simulink model "System_franare"  (R2020b)
settings: Solver=ode45  StartTime=0.0  StopTime=15  FixedStep=0.00001  RelTol=1e-3
values from neighbouring files (symbols this model uses):
  Ar = eval(Ar)    [liniarizare_hydraulic_stud.m]
  Br = eval(Br)    [liniarizare_hydraulic_stud.m]
  C = [1 0 0 0 0]    [liniarizare_hydraulic_stud.m]
  K = place(Ar,Br,[-99  -100  -101  -200  -201])    [liniarizare_hydraulic_stud.m]
  L = L'    [liniarizare_hydraulic_stud.m]
  N = -inv(C*inv(Ar-Br*K)*Br)    [liniarizare_hydraulic_stud.m]
undefined symbols (not defined in the file or in its folder): proces, proces2
libraries: simulink x1
settings Model: Creator=Zsofi  LastModifiedBy=tudor
settings DataIOCC: ReturnWorkspaceOutputs=off
settings DebuggingCC: ArithmeticOperatorsInVariantConditions=warning
settings SFSimCC: SimUseLocalCustomCode=off  CustomCodeUndefinedFunction=UseInterfaceOnly
settings RTWCC: RTWUseLocalCustomCode=off
settings CodeAppCC: StateflowObjectComments=on

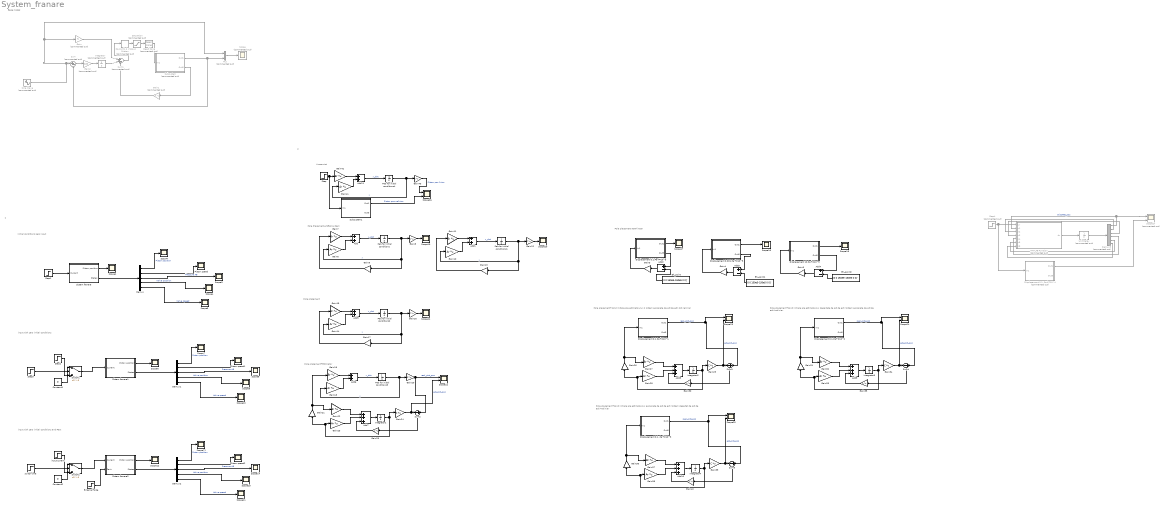
== system System_franare ==
  note: Linear sist
  note: Pole placement+cond initiale ale estimatorului si sistem apropiate de pct de ech sist neliniar
  note: 2
  note: Pole placement+Estimator
  note: Pole placement
  note: 1
  note: Pole Placement-LINEAR system
  note: input with zero initial conditions
  note: Initial conditions,zero input
  note: Base model
  note: input with zero initial conditions and Fext
  note: Pole placement NON-linear
  note: Pole placement+cond initiale ale estimatorului departate de pct de ech (sistem apropiate de pct de ech)-neliniar
  note: Pole placement+cond initiale ale estimatorului apropiate de pct de ech (sistem departat de pct de ech)-neliniar
  Add{,1,5..6,11} (5 alike) : Sum
  Add{7..10} (4 alike) : Sum  Inputs=+++
  Add2 : Sum  Inputs=+-
  Add3 : Sum  Inputs=+-
  Add4 : Sum  Inputs=+-
  Constant1 : Constant  Value=0
  Constant2 : Constant  Value=0
  Coulomb & Viscous Friction : simulink/Discontinuities/Coulomb & Viscous Friction  Commented=on  offset=0.005  gain=1
  DIsplacement 0.1,,Pa+=10^3 : Subsystem
  DIsplacement 0.1,,Pa+=10^4 : Subsystem  Commented=on
  DIsplacement 0.1,Pa+=10^1 : Subsystem
  DIsplacement 0.1,Pa+=10^2 : Subsystem
  DIsplacement 0.1,Pa+=10^5 : Subsystem
  Dead Zone : DeadZone  Commented=on  LowerValue=-0.005  UpperValue=0.005  SaturateOnIntegerOverflow=on
  Demux : Demux  Outputs=5
  Demux1 : Demux  Outputs=5
  Demux2 : Demux  Outputs=5
  Demux3 : Demux  Commented=on  Outputs=6
  Displacement 0.001,Pa+=10^5 : Subsystem
  Displacement 10,Pa+=10^5 : Subsystem
  Eh_point : Constant  Value=[0 0 150e5-150e5 0 0]'
  Eh_point1 : Constant  Value=[0 0 150e5-150e5 0 0]'
  Eh_point2 : Constant  Value=[0 0 150e5-150e5 0 0]'
  External force : Step  Time=6  After=300  SampleTime=0
  Gain : Gain  Commented=on  Gain=N
  Gain1 : Gain  Commented=on  Gain=K  Multiplication=Matrix(K*u)
  Gain{6,10,14,18,23,28,33,38,41} (9 alike) : Gain  Gain=Ar  Multiplication=Matrix(K*u)
  Gain{7,11,15,19,22,27,32,37,42} (9 alike) : Gain  Gain=Br  Multiplication=Matrix(K*u)
  Gain{8,12,16,20,24,29,34,39,43} (9 alike) : Gain  Gain=C  Multiplication=Matrix(K*u)
  Gain{3..5,9,13,17,21,26,31,36} (10 alike) : Gain  Gain=-K  Multiplication=Matrix(K*u)
  Gain2 : Gain  Commented=on  Gain=100
  Gain{25,30,35,40} (4 alike) : Gain  Gain=L  Multiplication=Matrix(K*u)
  Integrator : Integrator  Commented=on
  Integrator1 : Integrator
  Integrator2 : Integrator  InitialCondition=[0.01 0 0 0 0]'
  Integrator3 : Integrator  InitialCondition=[1 0 10e5 0 0]'
  Integrator4 : Integrator  InitialCondition=[0.4 0 1e5 0 0]'
  MATLAB Function : MATLAB Function  Commented=on  TreatAsAtomicUnit=on
  Mux : Mux  Commented=on  Inputs=2
  Pab for initial conditions : Integrator  InitialCondition=[0.1 0 1e5 0 0]
  Pab for initial conditions1 : Integrator  InitialCondition=[10 0 1e5 0 0]
  Pab for initial conditions2 : Integrator  InitialCondition=[0.1 0 1e5 0 0]
  Pab for initial conditions3 : Integrator  InitialCondition=[0.1 0 1e5 0 0]
  Pab for initial conditions4 : Integrator  InitialCondition=[0.001 0 0 0 0]
  Piston speed : Scope
  Piston speed1 : Scope
  Piston speed2 : Scope
  Saturation : Saturate  Commented=on  UpperLimit=0.1  LowerLimit=-0.1
  Scope : Scope  Commented=on
  Scope{1..21} (21 alike) : Scope
  Scope{22..26} (5 alike) : Scope  NumInputPorts=2
  Scope27 : Scope  Commented=on  NumInputPorts=2
  Sine Wave : Sin  Commented=on  Amplitude=0.02  Frequency=0.5  SampleTime=0
  Sistem franare : Subsystem
  Sistem franare1 : Subsystem
  Sistem franare2 : Subsystem
  Step : Step  Before=0.05  After=0  SampleTime=0
  Step1 : Step  Time=0  After=0  SampleTime=0
  Step2 : Step  Time=0  After=0.05  SampleTime=0
  Step3 : Step  SampleTime=0
  Step4 : Step  Commented=on  Time=0  After=0  SampleTime=0.00001
  Subsystem : Subsystem  Commented=on
  Subsystem1 : Subsystem
  Sum : Sum  Commented=on  Inputs=|+-
  Sum1 : Sum  Commented=on  Inputs=|++-
  Sum{2..5} (4 alike) : Sum  Inputs=-|+
  Switch1 : Switch  Criteria=u2 > Threshold
  Switch2 : Switch  Criteria=u2 > Threshold
  Unit Delay : UnitDelay  Commented=on  InitialCondition=[0.001 0 151e5 150e5 0 0]  SampleTime=-1  HasFrameUpgradeWarning=on
  input current : Step  Time=0  After=0.05  SampleTime=0
  switch time : Step  SampleTime=0
  wires:
  Subsystem/1(Out1) -> Mux/2, Sum/2
  Subsystem/2(Out3) -> Gain1/1
  Gain1/1 -> Sum1/3
  Sine Wave/1 -> Gain/1, Mux/1, Sum/1
  Gain/1 -> Sum1/1
  Sum/1 -> Gain2/1
  Gain2/1 -> Integrator/1
  Integrator/1 -> Sum1/2
  Mux/1 -> Scope/1
  Sum1/1 -> Coulomb & Viscous Friction/1
  Saturation/1 -> Dead Zone/1
  Dead Zone/1 -> Subsystem/1(In1)
  Coulomb & Viscous Friction/1 -> Saturation/1
  Sistem franare/1(Piston position) -> Scope1/1
  Sistem franare/2(States) -> Demux/1
  Demux/1 -> Scope2/1  "Piston position"
  Demux/2 -> Piston speed/1
  Demux/3 -> Scope3/1  "Pressure AB"
  Demux/4 -> Scope4/1  "Valve position"
  Demux/5 -> Scope5/1  "Valve speed"
  Step1/1 -> Sistem franare/1(Current)
  Step2/1 -> Switch1/3
  Demux1/2 -> Piston speed1/1
  Switch1/1 -> Sistem franare1/1(Current)
  Demux1/5 -> Scope10/1  "Valve speed"
  Sistem franare1/2(States) -> Demux1/1
  Demux1/4 -> Scope9/1  "Valve position"
  Constant1/1 -> Switch1/1
  Demux1/3 -> Scope8/1  "Pressure AB"
  Step3/1 -> Switch1/2
  Demux1/1 -> Scope7/1  "Piston position"
  Sistem franare1/1(Piston position) -> Scope6/1
  input current/1 -> Switch2/3
  Sistem franare2/2(States) -> Demux2/1
  Demux2/2 -> Piston speed2/1
  Switch2/1 -> Sistem franare2/1(Current)
  Demux2/5 -> Scope11/1  "Valve speed"
  Demux2/1 -> Scope13/1  "Piston position"
  Sistem franare2/1(Piston position) -> Scope12/1
  Constant2/1 -> Switch2/1
  Demux2/4 -> Scope15/1  "Valve position"
  switch time/1 -> Switch2/2
  Demux2/3 -> Scope14/1  "Pressure AB"
  External force/1 -> Sistem franare2/2(Fext)
  Displacement 0.001,Pa+=10^5/1(Out1) -> Scope16/1
  Gain4/1 -> Displacement 0.001,Pa+=10^5/1(In1)
  DIsplacement 0.1,Pa+=10^5/1(Out1) -> Scope17/1
  Gain3/1 -> DIsplacement 0.1,Pa+=10^5/1(In1)
  Displacement 10,Pa+=10^5/1(Out1) -> Scope18/1
  Gain5/1 -> Displacement 10,Pa+=10^5/1(In1)
  Pab for initial conditions/1 -> Gain8/1, Gain9/1, Gain6/1  "x"
  Gain6/1 -> Add/2
  Gain7/1 -> Add/1
  Add/1 -> Pab for initial conditions/1  "x_dot"
  Gain9/1 -> Gain7/1
  Gain8/1 -> Scope19/1
  Gain10/1 -> Add1/2
  Add1/1 -> Pab for initial conditions1/1  "x_dot"
  Gain13/1 -> Gain11/1
  Pab for initial conditions1/1 -> Gain12/1, Gain13/1, Gain10/1  "x"
  Gain11/1 -> Add1/1
  Gain12/1 -> Scope20/1
  Add2/1 -> Gain3/1
  DIsplacement 0.1,Pa+=10^5/2(Out3) -> Add2/1
  Eh_point/1 -> Add2/2
  Displacement 0.001,Pa+=10^5/2(Out3) -> Add3/1
  Eh_point1/1 -> Add3/2
  Add3/1 -> Gain4/1
  Displacement 10,Pa+=10^5/2(Out3) -> Add4/1
  Add4/1 -> Gain5/1
  Eh_point2/1 -> Add4/2
  Gain15/1 -> Add5/1
  Add5/1 -> Pab for initial conditions2/1  "x_dot"
  Gain16/1 -> Scope21/1
  Gain17/1 -> Gain15/1
  Gain14/1 -> Add5/2
  Pab for initial conditions2/1 -> Gain16/1, Gain17/1, Gain14/1  "x"
  Gain19/1 -> Add6/1
  Add6/1 -> Pab for initial conditions3/1  "x_dot"
  Gain20/1 -> Sum2/2, Scope22/1  "real_pist_pos"
  Gain21/1 -> Gain22/1, Gain19/1
  Gain18/1 -> Add6/2
  Pab for initial conditions3/1 -> Gain20/1, Gain18/1  "x"
  Gain23/1 -> Add7/2
  Gain22/1 -> Add7/1
  Gain24/1 -> Scope22/2, Sum2/1  "est_pist_pos"
  Add7/1 -> Integrator1/1
  Integrator1/1 -> Gain24/1, Gain21/1, Gain23/1
  Sum2/1 -> Gain25/1
  Gain25/1 -> Add7/3
  Sum3/1 -> Gain30/1
  Gain29/1 -> Scope23/2, Sum3/1  "est_pist_pos"
  Gain28/1 -> Add8/2
  Add8/1 -> Integrator2/1
  Gain30/1 -> Add8/3
  Gain27/1 -> Add8/1
  Gain26/1 -> DIsplacement 0.1,Pa+=10^1/1(In1), Gain27/1
  Integrator2/1 -> Gain29/1, Gain26/1, Gain28/1
  DIsplacement 0.1,Pa+=10^1/1(Out1) -> Scope23/1, Sum3/2  "real_pist_pos"
  DIsplacement 0.1,Pa+=10^2/1(Out1) -> Scope24/1, Sum4/2  "real_pist_pos"
  Gain35/1 -> Add9/3
  Gain32/1 -> Add9/1
  Gain31/1 -> DIsplacement 0.1,Pa+=10^2/1(In1), Gain32/1
  Gain33/1 -> Add9/2
  Add9/1 -> Integrator3/1
  Sum4/1 -> Gain35/1
  Integrator3/1 -> Gain34/1, Gain31/1, Gain33/1
  Gain34/1 -> Scope24/2, Sum4/1  "est_pist_pos"
  Gain39/1 -> Scope25/2, Sum5/1  "est_pist_pos"
  Integrator4/1 -> Gain39/1, Gain36/1, Gain38/1
  Gain38/1 -> Add10/2
  Sum5/1 -> Gain40/1
  Gain36/1 -> DIsplacement 0.1,,Pa+=10^3/1(In1), Gain37/1
  Gain40/1 -> Add10/3
  Add10/1 -> Integrator4/1
  DIsplacement 0.1,,Pa+=10^3/1(Out1) -> Scope25/1, Sum5/2  "real_pist_pos"
  Gain37/1 -> Add10/1
  Add11/1 -> Pab for initial conditions4/1  "x_dot"
  Gain41/1 -> Add11/2
  Pab for initial conditions4/1 -> Gain41/1, Gain43/1  "x"
  Gain42/1 -> Add11/1
  Step/1 -> Subsystem1/1(In1), Gain42/1
  Gain43/1 -> Scope26/1  "Piston pos liniar"
  Subsystem1/1(Out1) -> Scope26/2  "Piston pos neliniar"
  DIsplacement 0.1,,Pa+=10^4/1(Out1) -> Scope27/2
  Unit Delay/1 -> Demux3/1
  Demux3/1 -> Scope27/1, MATLAB Function/2(x1)  "Discrete_pos"
  Demux3/5 -> MATLAB Function/6(x5)
  Demux3/6 -> MATLAB Function/7(x6)
  Step4/1 -> DIsplacement 0.1,,Pa+=10^4/1(In1), MATLAB Function/1(uv)
  Demux3/3 -> MATLAB Function/4(x3)
  Demux3/4 -> MATLAB Function/5(x4)
  Demux3/2 -> MATLAB Function/3(x2)
  MATLAB Function/1(dx) -> Unit Delay/1

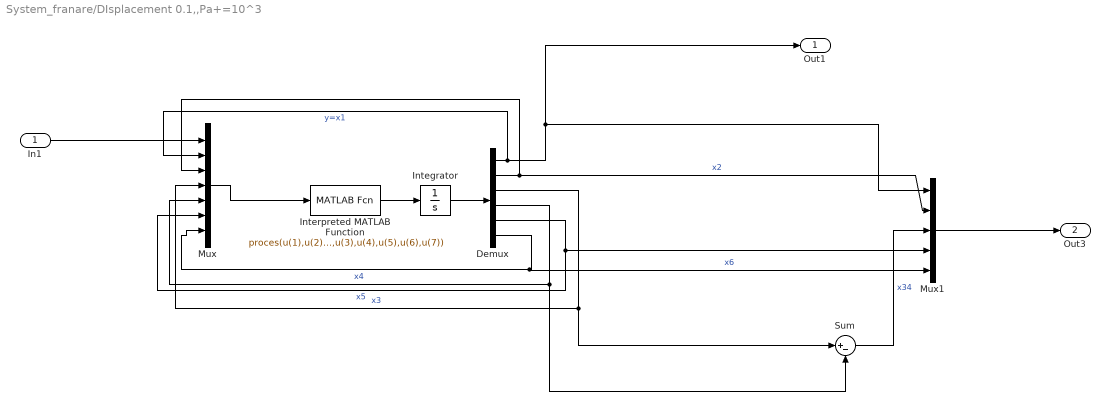
== system System_franare/DIsplacement 0.1,,Pa+=10^3 ==
  In1 : Inport
  Demux : Demux  Outputs=6
  Integrator : Integrator  InitialCondition=[1 0 150e5 150e5 0 0]
  Interpreted MATLAB Function : MATLABFcn  MATLABFcn=proces(u(1),u(2),u(3),u(4),u(5),u(6),u(7))  OutputSignalType=real  Output1D=off
  Mux : Mux  Inputs=7
  Mux1 : Mux  Inputs=5
  Sum : Sum  Inputs=|+-
  Out1 : Outport
  Out3 : Outport  Port=2
  wires:
  Demux/4 -> Sum/2, Mux/5  "x4"
  Demux/3 -> Sum/1, Mux/4  "x3"
  Demux/6 -> Mux1/5, Mux/7  "x6"
  Demux/5 -> Mux/6, Mux1/4  "x5"
  Demux/1 -> Mux/2, Out1/1, Mux1/1  "y=x1"
  Demux/2 -> Mux1/2, Mux/3  "x2"
  Interpreted MATLAB Function/1 -> Integrator/1
  In1/1 -> Mux/1
  Sum/1 -> Mux1/3  "x34"
  Integrator/1 -> Demux/1
  Mux1/1 -> Out3/1
  Mux/1 -> Interpreted MATLAB Function/1

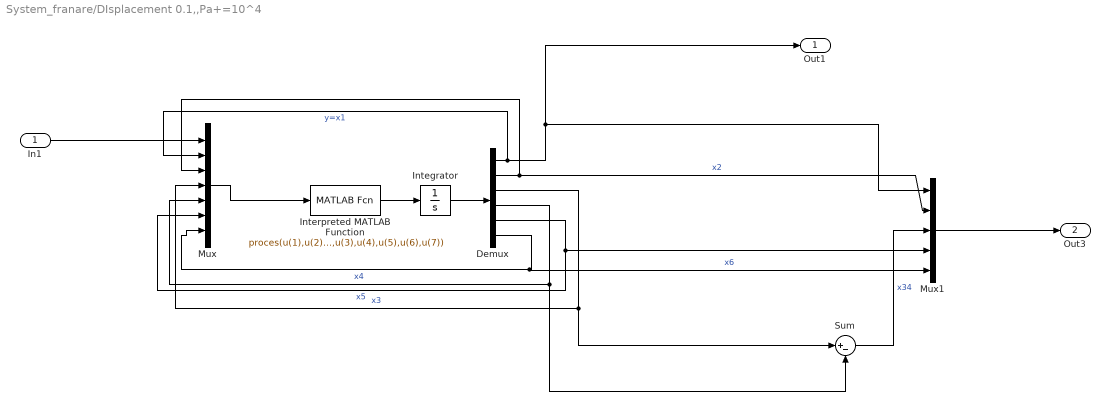
== system System_franare/DIsplacement 0.1,,Pa+=10^4 ==
  In1 : Inport
  Demux : Demux  Outputs=6
  Integrator : Integrator  InitialCondition=[0.001 0 151e5 150e5 0 0]
  Interpreted MATLAB Function : MATLABFcn  MATLABFcn=proces(u(1),u(2),u(3),u(4),u(5),u(6),u(7))  OutputSignalType=real  Output1D=off
  Mux : Mux  Inputs=7
  Mux1 : Mux  Inputs=5
  Sum : Sum  Inputs=|+-
  Out1 : Outport
  Out3 : Outport  Port=2
  wires:
  Demux/4 -> Sum/2, Mux/5  "x4"
  Demux/3 -> Sum/1, Mux/4  "x3"
  Demux/6 -> Mux1/5, Mux/7  "x6"
  Demux/5 -> Mux/6, Mux1/4  "x5"
  Demux/1 -> Mux/2, Out1/1, Mux1/1  "y=x1"
  Demux/2 -> Mux1/2, Mux/3  "x2"
  Interpreted MATLAB Function/1 -> Integrator/1
  In1/1 -> Mux/1
  Sum/1 -> Mux1/3  "x34"
  Integrator/1 -> Demux/1
  Mux1/1 -> Out3/1
  Mux/1 -> Interpreted MATLAB Function/1

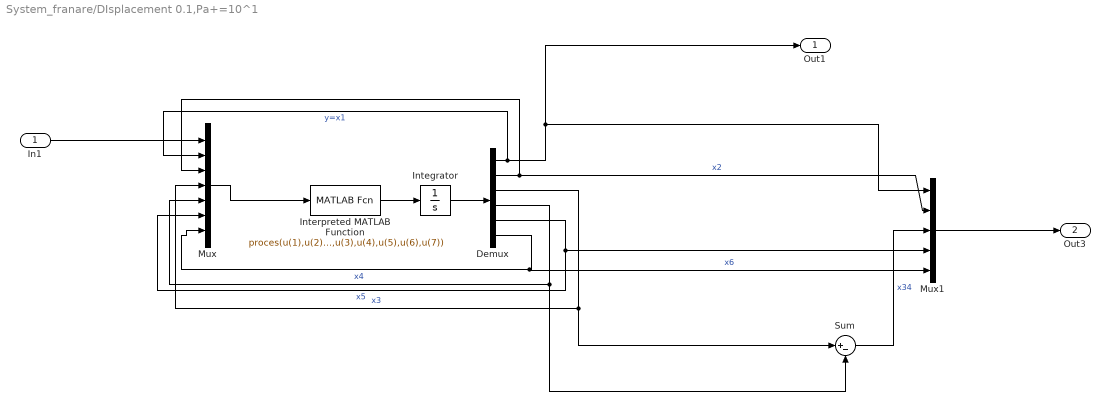
== system System_franare/DIsplacement 0.1,Pa+=10^1 ==
  In1 : Inport
  Demux : Demux  Outputs=6
  Integrator : Integrator  InitialCondition=[0.01 0 151e5 150e5 0 0]
  Interpreted MATLAB Function : MATLABFcn  MATLABFcn=proces(u(1),u(2),u(3),u(4),u(5),u(6),u(7))  OutputSignalType=real  Output1D=off
  Mux : Mux  Inputs=7
  Mux1 : Mux  Inputs=5
  Sum : Sum  Inputs=|+-
  Out1 : Outport
  Out3 : Outport  Port=2
  wires:
  Demux/4 -> Sum/2, Mux/5  "x4"
  Demux/3 -> Sum/1, Mux/4  "x3"
  Demux/6 -> Mux1/5, Mux/7  "x6"
  Demux/5 -> Mux/6, Mux1/4  "x5"
  Demux/1 -> Mux/2, Out1/1, Mux1/1  "y=x1"
  Demux/2 -> Mux1/2, Mux/3  "x2"
  Interpreted MATLAB Function/1 -> Integrator/1
  In1/1 -> Mux/1
  Sum/1 -> Mux1/3  "x34"
  Integrator/1 -> Demux/1
  Mux1/1 -> Out3/1
  Mux/1 -> Interpreted MATLAB Function/1

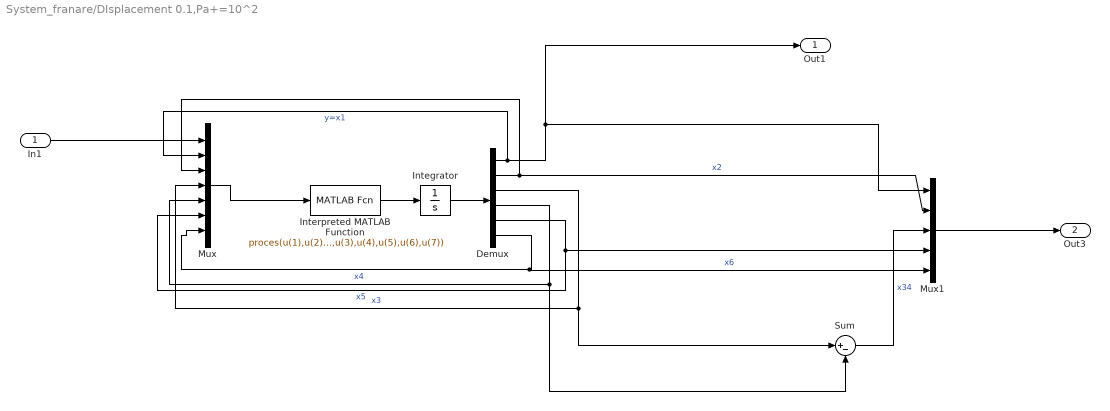
== system System_franare/DIsplacement 0.1,Pa+=10^2 ==
  In1 : Inport
  Demux : Demux  Outputs=6
  Integrator : Integrator  InitialCondition=[0.001 0 150e5 150e5 0 0]
  Interpreted MATLAB Function : MATLABFcn  MATLABFcn=proces(u(1),u(2),u(3),u(4),u(5),u(6),u(7))  OutputSignalType=real  Output1D=off
  Mux : Mux  Inputs=7
  Mux1 : Mux  Inputs=5
  Sum : Sum  Inputs=|+-
  Out1 : Outport
  Out3 : Outport  Port=2
  wires:
  Demux/4 -> Sum/2, Mux/5  "x4"
  Demux/3 -> Sum/1, Mux/4  "x3"
  Demux/6 -> Mux1/5, Mux/7  "x6"
  Demux/5 -> Mux/6, Mux1/4  "x5"
  Demux/1 -> Mux/2, Out1/1, Mux1/1  "y=x1"
  Demux/2 -> Mux1/2, Mux/3  "x2"
  Interpreted MATLAB Function/1 -> Integrator/1
  In1/1 -> Mux/1
  Sum/1 -> Mux1/3  "x34"
  Integrator/1 -> Demux/1
  Mux1/1 -> Out3/1
  Mux/1 -> Interpreted MATLAB Function/1

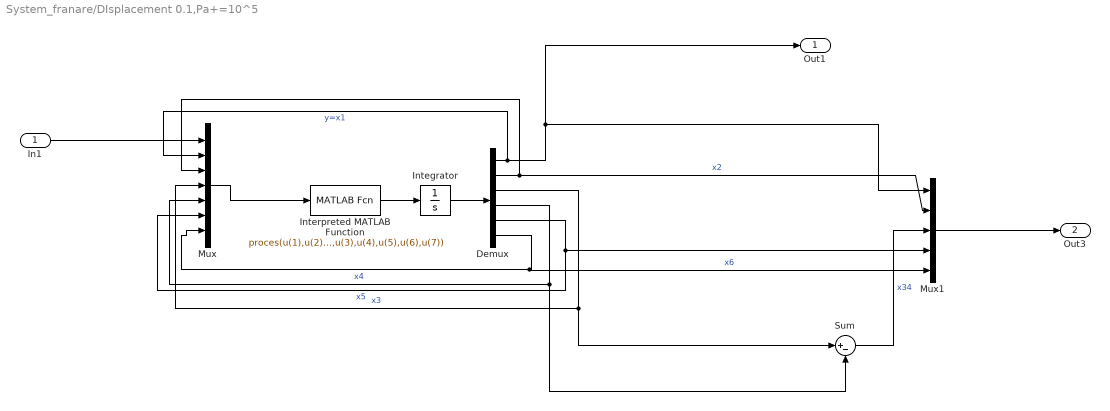
== system System_franare/DIsplacement 0.1,Pa+=10^5 ==
  In1 : Inport
  Demux : Demux  Outputs=6
  Integrator : Integrator  InitialCondition=[0.1 0 151e5 150e5 0 0]
  Interpreted MATLAB Function : MATLABFcn  MATLABFcn=proces(u(1),u(2),u(3),u(4),u(5),u(6),u(7))  OutputSignalType=real  Output1D=off
  Mux : Mux  Inputs=7
  Mux1 : Mux  Inputs=5
  Sum : Sum  Inputs=|+-
  Out1 : Outport
  Out3 : Outport  Port=2
  wires:
  Demux/4 -> Sum/2, Mux/5  "x4"
  Demux/3 -> Sum/1, Mux/4  "x3"
  Demux/6 -> Mux1/5, Mux/7  "x6"
  Demux/5 -> Mux/6, Mux1/4  "x5"
  Demux/1 -> Mux/2, Out1/1, Mux1/1  "y=x1"
  Demux/2 -> Mux1/2, Mux/3  "x2"
  Interpreted MATLAB Function/1 -> Integrator/1
  In1/1 -> Mux/1
  Sum/1 -> Mux1/3  "x34"
  Integrator/1 -> Demux/1
  Mux1/1 -> Out3/1
  Mux/1 -> Interpreted MATLAB Function/1

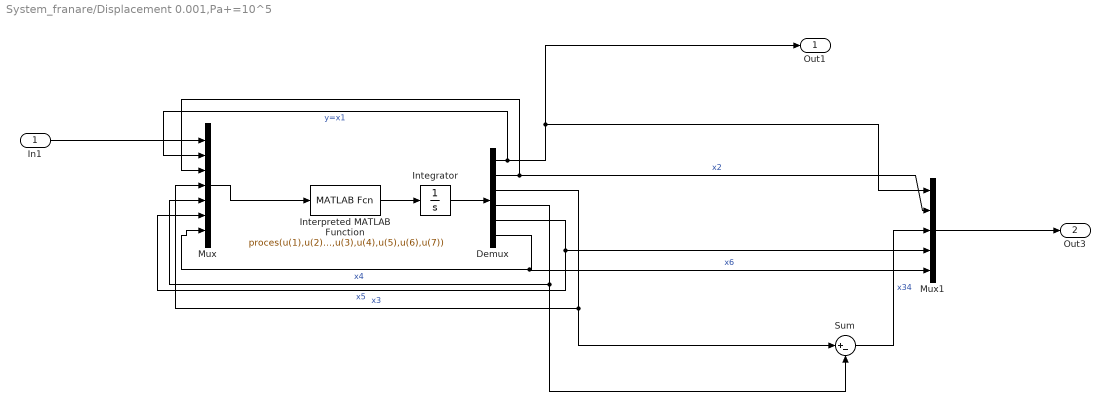
== system System_franare/Displacement 0.001,Pa+=10^5 ==
  In1 : Inport
  Demux : Demux  Outputs=6
  Integrator : Integrator  InitialCondition=[0.001 0 151e5 150e5 0 0]
  Interpreted MATLAB Function : MATLABFcn  MATLABFcn=proces(u(1),u(2),u(3),u(4),u(5),u(6),u(7))  OutputSignalType=real  Output1D=off
  Mux : Mux  Inputs=7
  Mux1 : Mux  Inputs=5
  Sum : Sum  Inputs=|+-
  Out1 : Outport
  Out3 : Outport  Port=2
  wires:
  Demux/4 -> Sum/2, Mux/5  "x4"
  Demux/3 -> Sum/1, Mux/4  "x3"
  Demux/6 -> Mux1/5, Mux/7  "x6"
  Demux/5 -> Mux/6, Mux1/4  "x5"
  Demux/1 -> Mux/2, Out1/1, Mux1/1  "y=x1"
  Demux/2 -> Mux1/2, Mux/3  "x2"
  Interpreted MATLAB Function/1 -> Integrator/1
  In1/1 -> Mux/1
  Sum/1 -> Mux1/3  "x34"
  Integrator/1 -> Demux/1
  Mux1/1 -> Out3/1
  Mux/1 -> Interpreted MATLAB Function/1

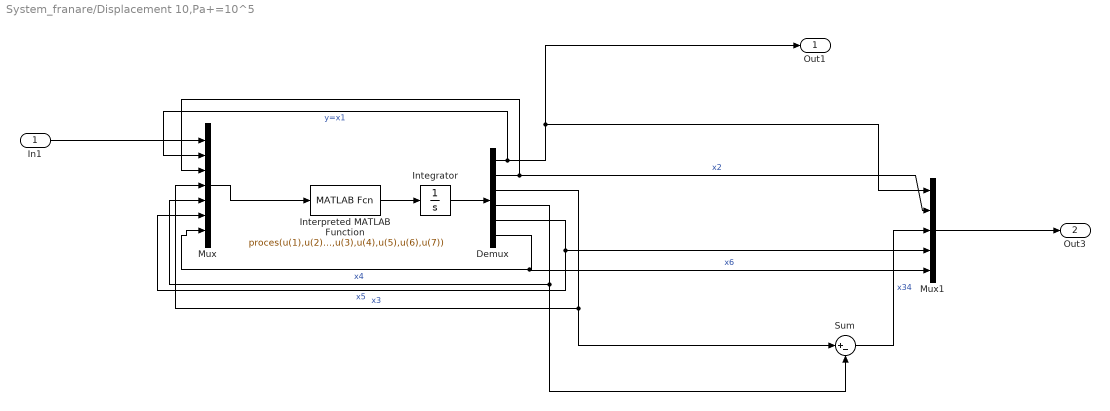
== system System_franare/Displacement 10,Pa+=10^5 ==
  In1 : Inport
  Demux : Demux  Outputs=6
  Integrator : Integrator  InitialCondition=[10 0 150e5 151e5 0 0]
  Interpreted MATLAB Function : MATLABFcn  MATLABFcn=proces(u(1),u(2),u(3),u(4),u(5),u(6),u(7))  OutputSignalType=real  Output1D=off
  Mux : Mux  Inputs=7
  Mux1 : Mux  Inputs=5
  Sum : Sum  Inputs=|+-
  Out1 : Outport
  Out3 : Outport  Port=2
  wires:
  Demux/4 -> Sum/2, Mux/5  "x4"
  Demux/3 -> Sum/1, Mux/4  "x3"
  Demux/6 -> Mux1/5, Mux/7  "x6"
  Demux/5 -> Mux/6, Mux1/4  "x5"
  Demux/1 -> Mux/2, Out1/1, Mux1/1  "y=x1"
  Demux/2 -> Mux1/2, Mux/3  "x2"
  Interpreted MATLAB Function/1 -> Integrator/1
  In1/1 -> Mux/1
  Sum/1 -> Mux1/3  "x34"
  Integrator/1 -> Demux/1
  Mux1/1 -> Out3/1
  Mux/1 -> Interpreted MATLAB Function/1

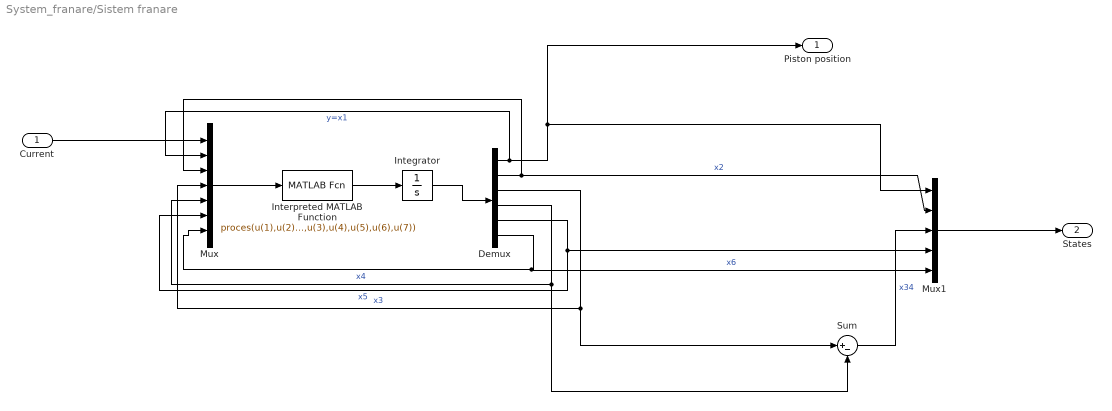
== system System_franare/Sistem franare ==
  Current : Inport
  Demux : Demux  Outputs=6
  Integrator : Integrator  InitialCondition=[0.01 0 10000 10 0.05 0]
  Interpreted MATLAB Function : MATLABFcn  MATLABFcn=proces(u(1),u(2),u(3),u(4),u(5),u(6),u(7))  OutputSignalType=real  Output1D=off
  Mux : Mux  Inputs=7
  Mux1 : Mux  Inputs=5
  Sum : Sum  Inputs=|+-
  Piston position : Outport
  States : Outport  Port=2
  wires:
  Demux/4 -> Sum/2, Mux/5  "x4"
  Demux/3 -> Sum/1, Mux/4  "x3"
  Demux/6 -> Mux1/5, Mux/7  "x6"
  Demux/5 -> Mux/6, Mux1/4  "x5"
  Demux/1 -> Mux/2, Piston position/1, Mux1/1  "y=x1"
  Demux/2 -> Mux1/2, Mux/3  "x2"
  Interpreted MATLAB Function/1 -> Integrator/1
  Mux/1 -> Interpreted MATLAB Function/1
  Current/1 -> Mux/1
  Sum/1 -> Mux1/3  "x34"
  Integrator/1 -> Demux/1
  Mux1/1 -> States/1

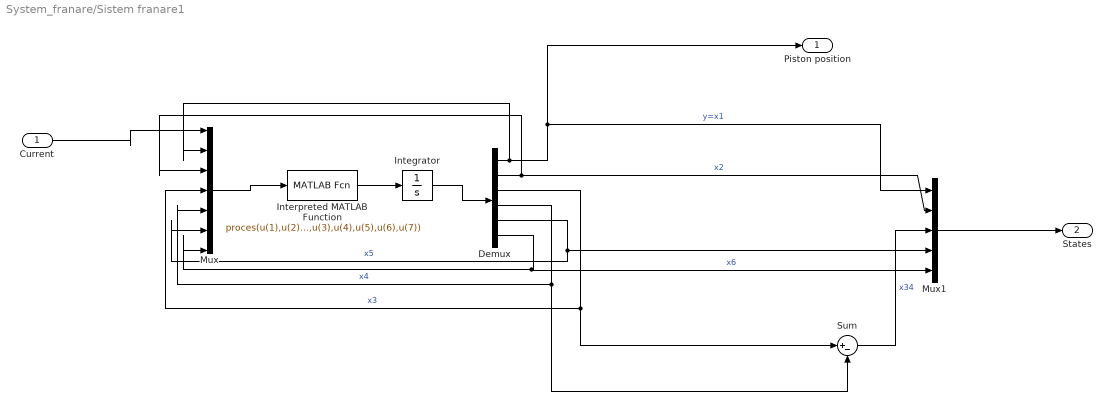
== system System_franare/Sistem franare1 ==
  Current : Inport
  Demux : Demux  Outputs=6
  Integrator : Integrator
  Interpreted MATLAB Function : MATLABFcn  MATLABFcn=proces(u(1),u(2),u(3),u(4),u(5),u(6),u(7))  OutputSignalType=real  Output1D=off
  Mux : Mux  Inputs=7
  Mux1 : Mux  Inputs=5
  Sum : Sum  Inputs=|+-
  Piston position : Outport
  States : Outport  Port=2
  wires:
  Demux/4 -> Sum/2, Mux/5  "x4"
  Demux/3 -> Sum/1, Mux/4  "x3"
  Demux/6 -> Mux1/5, Mux/7  "x6"
  Demux/5 -> Mux/6, Mux1/4  "x5"
  Demux/1 -> Mux/2, Piston position/1, Mux1/1  "y=x1"
  Demux/2 -> Mux1/2, Mux/3  "x2"
  Interpreted MATLAB Function/1 -> Integrator/1
  Mux/1 -> Interpreted MATLAB Function/1
  Current/1 -> Mux/1
  Sum/1 -> Mux1/3  "x34"
  Integrator/1 -> Demux/1
  Mux1/1 -> States/1

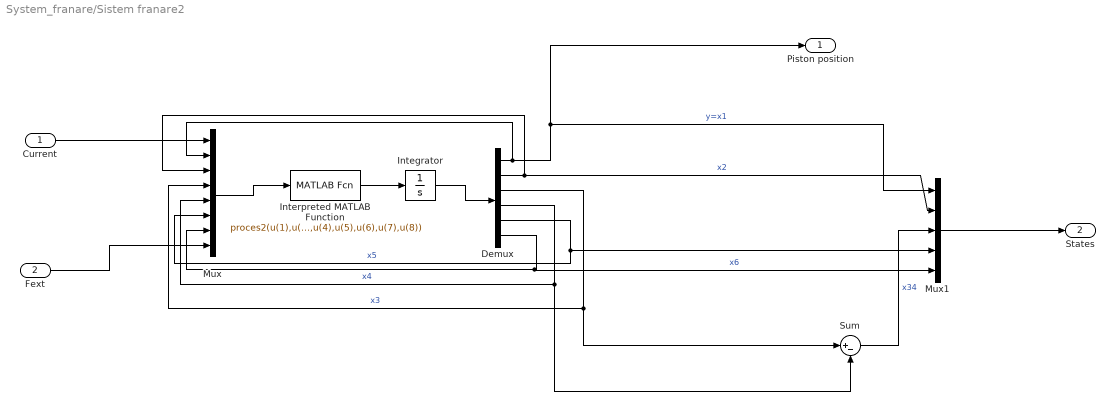
== system System_franare/Sistem franare2 ==
  Current : Inport
  Fext : Inport  Port=2
  Demux : Demux  Outputs=6
  Integrator : Integrator
  Interpreted MATLAB Function : MATLABFcn  MATLABFcn=proces2(u(1),u(2),u(3),u(4),u(5),u(6),u(7),u(8))  OutputSignalType=real  Output1D=off
  Mux : Mux  Inputs=8
  Mux1 : Mux  Inputs=5
  Sum : Sum  Inputs=|+-
  Piston position : Outport
  States : Outport  Port=2
  wires:
  Demux/4 -> Sum/2, Mux/5  "x4"
  Demux/3 -> Sum/1, Mux/4  "x3"
  Demux/6 -> Mux1/5, Mux/7  "x6"
  Demux/5 -> Mux/6, Mux1/4  "x5"
  Demux/1 -> Mux/2, Piston position/1, Mux1/1  "y=x1"
  Demux/2 -> Mux1/2, Mux/3  "x2"
  Interpreted MATLAB Function/1 -> Integrator/1
  Mux/1 -> Interpreted MATLAB Function/1
  Current/1 -> Mux/1
  Sum/1 -> Mux1/3  "x34"
  Integrator/1 -> Demux/1
  Mux1/1 -> States/1
  Fext/1 -> Mux/8

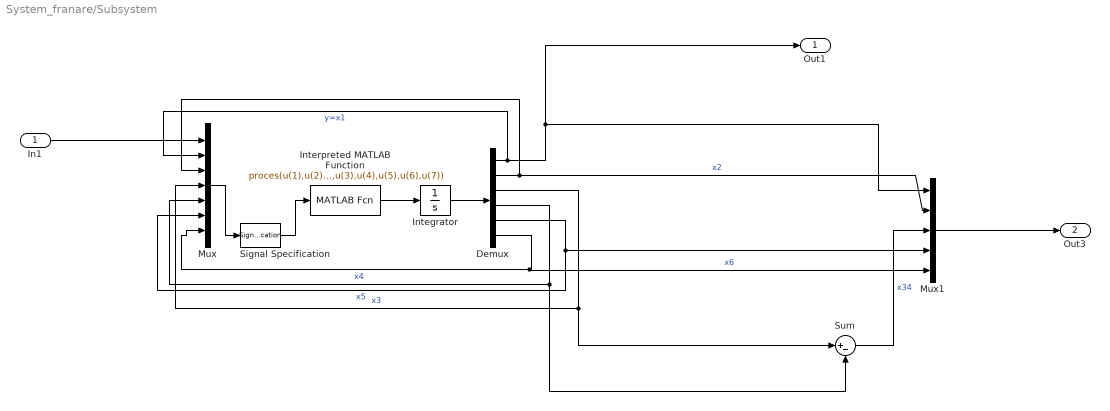
== system System_franare/Subsystem ==
  In1 : Inport
  Demux : Demux  Outputs=6
  Integrator : Integrator
  Interpreted MATLAB Function : MATLABFcn  MATLABFcn=proces(u(1),u(2),u(3),u(4),u(5),u(6),u(7))  OutputSignalType=real  Output1D=off
  Mux : Mux  Inputs=7
  Mux1 : Mux  Inputs=5
  Signal Specification : SignalSpecification  Dimensions=[1,7]
  Sum : Sum  Inputs=|+-
  Out1 : Outport
  Out3 : Outport  Port=2
  wires:
  Demux/4 -> Sum/2, Mux/5  "x4"
  Demux/3 -> Sum/1, Mux/4  "x3"
  Demux/6 -> Mux1/5, Mux/7  "x6"
  Demux/5 -> Mux/6, Mux1/4  "x5"
  Demux/1 -> Mux/2, Out1/1, Mux1/1  "y=x1"
  Demux/2 -> Mux1/2, Mux/3  "x2"
  Interpreted MATLAB Function/1 -> Integrator/1
  Mux/1 -> Signal Specification/1
  In1/1 -> Mux/1
  Sum/1 -> Mux1/3  "x34"
  Integrator/1 -> Demux/1
  Mux1/1 -> Out3/1
  Signal Specification/1 -> Interpreted MATLAB Function/1

== system System_franare/Subsystem1 ==
  In1 : Inport
  Demux : Demux  Outputs=6
  Integrator : Integrator  InitialCondition=[0.001 0 150e5 150e5 0 0]
  Interpreted MATLAB Function : MATLABFcn  MATLABFcn=proces(u(1),u(2),u(3),u(4),u(5),u(6),u(7))  OutputSignalType=real  Output1D=off
  Mux : Mux  Inputs=7
  Mux1 : Mux  Inputs=5
  Sum : Sum  Inputs=|+-
  Out1 : Outport
  Out3 : Outport  Port=2
  wires:
  Demux/4 -> Sum/2, Mux/5  "x4"
  Demux/3 -> Sum/1, Mux/4  "x3"
  Demux/6 -> Mux1/5, Mux/7  "x6"
  Demux/5 -> Mux/6, Mux1/4  "x5"
  Demux/1 -> Mux/2, Out1/1, Mux1/1  "y=x1"
  Demux/2 -> Mux1/2, Mux/3  "x2"
  Interpreted MATLAB Function/1 -> Integrator/1
  In1/1 -> Mux/1
  Sum/1 -> Mux1/3  "x34"
  Integrator/1 -> Demux/1
  Mux1/1 -> Out3/1
  Mux/1 -> Interpreted MATLAB Function/1

== matlab function System_franare/MATLAB Function ==
  data: uv input; dx output; x1 input; x2 input; x3 input; x4 input; x5 input; x6 input
function dx = fcn(uv,x1,x2,x3,x4,x5,x6)

% max control curent 0.1 A
% min control curent 0.005 A
Kv=0.001 ;%valve input coef - uv is a current (A)
%inputs
Fext=0;%***************
u1=Kv*uv; 
u2=Fext;
%experimental friction parameters from Hydraulic servo systems Springer
sigma=200;%N s/m
Fc0=50;%N
Fs0=25;%N
cs=0.011;% m/s
%de Silva article
Mt=32.7;%kg
Vh=8.9*10^(-5);% m
A1=1.14*10^(-3);%m^2
A2=0.633*10^(-3);%m^2
Ap=(A1+A2)/2;
%Slidning mode control of hydraulic systems
Ps=300*10^5;%Pa
Pt=1*10^5;%Pa
% other sources
E=1.7*10^6;% Pa
%valve dynamics FitzSimons and Palazzolo
wv=730;%Hz natural frequency
Dv=0.4;%damping
Fhs=0;%ignore internal valve friction
cv1=6.6043*10^(-4);%m^2/(s sqrt(Pa)) valve discharge coefficients
cv2=cv1;
cv3=cv1;
cv4=cv1;
% piston length l=0.05 m +> xmax/xmin este +-0.025 m

%Per de esantionare
Te=0.00001;

Ff=(sigma*x2+sign(x2)*(Fc0+Fs0*exp(-abs(x2)/cs)));
%Ff=sigma*x2;% linear friction
%Ff=0;
qA=(cv1*sg(x5)*sign(Ps-x3)*sqrt(abs(Ps-x3))-cv2*sg(-x5)*sign(x3-Pt)*sqrt(abs(x3-Pt)));
qB=(cv3*sg(-x5)*sign(Ps-x4)*sqrt(abs(Ps-x4))-cv4*sg(x5)*sign(x4-Pt)*sqrt(abs(x4-Pt)));

dx1=x1+Te*x2;
dx2=x2+Te*((x3-x4)*Ap-Ff-u2)/Mt;
dx3=x3+Te*(qA-Ap*x2)*E/(Vh+Ap*x1);
dx4=x4+Te*(qB+Ap*x2)*E/(Vh-Ap*x1);
dx5=x5+Te*x6;
dx6=x6+Te*wv^2*(u1-2*Dv/wv*x6-x5-Fhs*sign(x5));

dx=[dx1 dx2 dx3 dx4 dx5 dx6];

y = dx;
